simulink model "MPC_AVC"  (Simulink 8.5)
settings: Solver=ode5  StartTime=0.0  StopTime=4  FixedStep=dt  RelTol=1e-3
values from neighbouring files (symbols this model uses):
  A = F    [DMPC_AVC.m]    (also in Load_before.mat = [-209.443458109 -450.728478794 0 0 0 0 450.728478794 -209.44; Load_before_luan.mat = [-1.51362295222 -97.5366784553 0 0 0 0 95.8379605832 -0.9182)
  A_cons = [L_m;-L_m]    [DMPC_AVC.m]
  B = G    [DMPC_AVC.m]    (also in Load_before.mat = [-9.64474367822  2.65660382188; -7.76311006326  -5.616131872; Load_before_luan.mat = [-0.368065493108  -0.262854319087; -0.0702861565304  -0.0199)
  Bg = Bg(:,1:2)    [DMPC_AVC.m]
  C = H    [DMPC_AVC.m]    (also in Load_before.mat = [1.88477251669 -1.14284793707 5.77230310808 47.9525873536 -5; Load_before_luan.mat = [-15.8723139253 -1.67390261755 -0.939173865751 -0.9779387082)
  coefs = coefs(1,2:end)    [DMPC_AVC.m]
  dt = 0.00025    [DMPC_AVC.m]
  Hg = Bg(:,3)    [DMPC_AVC.m]
  L1 = dlqr(A',C',1e-5*eye(size(A)),1e-7)'    [DMPC_AVC.m]
  L2 = place(A',C',[0 0.1 -0.1 0.2 -0.2 0.3 -0.3 -0.4])    [DMPC_AVC.m]
  Lf = Kalman_Gain(A,C,Qf,Rf,Pf,Nsim,nout)    [DMPC_AVC.m]
  u_bound = [u_max;-u_min]    [DMPC_AVC.m]
undefined symbols (not defined in the file or in its folder): Ag, Cg, L_m, omega, psi
settings Model: Creator=Farhang  LastModifiedBy=p4wp4w
settings DebuggingCC: SolverPrmCheckMsg=warning  FcnCallInpInsideContextMsg=UseLocalSettings

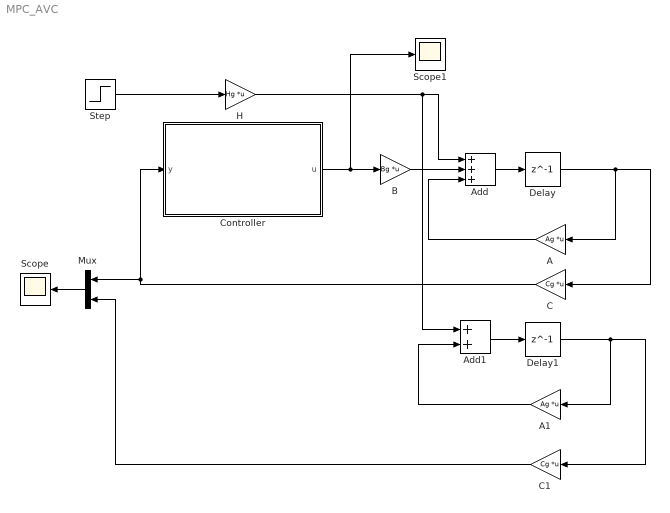
== system MPC_AVC ==
  A : Gain  Gain=Ag  Multiplication=Matrix(K*u)
  A1 : Gain  Gain=Ag  Multiplication=Matrix(K*u)
  Add : Sum  Inputs=+++
  Add1 : Sum
  B : Gain  Gain=Bg  Multiplication=Matrix(K*u)
  C : Gain  Gain=Cg  Multiplication=Matrix(K*u)
  C1 : Gain  Gain=Cg  Multiplication=Matrix(K*u)
  Controller : Subsystem
  Delay : Delay  DelayLength=1  InitialCondition=0
  Delay1 : Delay  DelayLength=1  InitialCondition=0
  H : Gain  Gain=Hg  Multiplication=Matrix(K*u)
  Mux : Mux  Inputs=2
  Scope : Scope
      settings: ShowLegends=on  YMin=-0.06  YMax=6.93889e-18
  Scope1 : Scope
      settings: ShowLegends=on  YMin=-0.0005  YMax=0.00055  SaveName=ScopeData2
  Step : Step  Time=2*dt  Before=1  After=0  SampleTime=0
  wires:
  Delay/1 -> A/1, C/1
  Controller/1(u) -> Scope1/1, B/1
  Add/1 -> Delay/1
  C/1 -> Mux/1, Controller/1(y)
  B/1 -> Add/2
  A/1 -> Add/3
  H/1 -> Add1/1, Add/1
  Step/1 -> H/1
  Delay1/1 -> C1/1, A1/1
  Add1/1 -> Delay1/1
  A1/1 -> Add1/2
  Mux/1 -> Scope/1
  C1/1 -> Mux/2

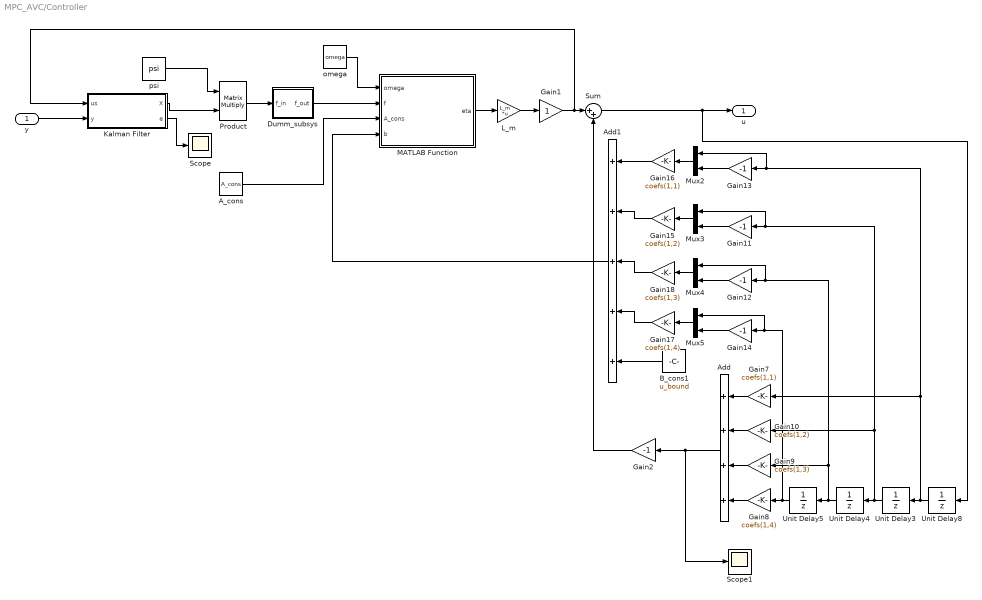
== system MPC_AVC/Controller ==
  y : Inport
  A_cons : Constant  Value=A_cons  SampleTime=dt
  Add : Sum  Inputs=++++
  Add1 : Sum  Inputs=+++++
  B_cons1 : Constant  Value=u_bound
  Dumm_subsys : Subsystem
  Gain1 : Gain
  Gain10 : Gain  Gain=coefs(1,2)
  Gain{2,11..14} (5 alike) : Gain  Gain=-1
  Gain15 : Gain  Gain=coefs(1,2)
  Gain16 : Gain  Gain=coefs(1,1)
  Gain17 : Gain  Gain=coefs(1,4)
  Gain18 : Gain  Gain=coefs(1,3)
  Gain7 : Gain  Gain=coefs(1,1)
  Gain8 : Gain  Gain=coefs(1,4)
  Gain9 : Gain  Gain=coefs(1,3)
  Kalman Filter : Subsystem  TreatAsAtomicUnit=on
  L_m : Gain  Gain=L_m  Multiplication=Matrix(K*u)
  MATLAB Function : MATLAB Function  TreatAsAtomicUnit=on
  Mux{2..5} (4 alike) : Mux  Inputs=2
  Product : Product  Multiplication=Matrix(*)  RndMeth=Zero
  Scope : Scope
      settings: YMin=-0.000155  YMax=-6.5e-05
  Scope1 : Scope
      settings: YMin=-0.00225  YMax=0.00225  SaveName=ScopeData3
  Sum : Sum  Inputs=|++
  Unit Delay{3..5,8} (4 alike) : UnitDelay  SampleTime=dt
  omega : Constant  Value=omega  SampleTime=dt
  psi : Constant  Value=psi  SampleTime=dt
  u : Outport
  wires:
  MATLAB Function/1(eta) -> L_m/1
  L_m/1 -> Gain1/1
  omega/1 -> MATLAB Function/1(omega)
  A_cons/1 -> MATLAB Function/3(A_cons)
  psi/1 -> Product/1
  y/1 -> Kalman Filter/2(y)
  Unit Delay8/1 -> Mux2/1, Gain13/1, Gain7/1, Unit Delay3/1
  Unit Delay3/1 -> Mux3/1, Gain11/1, Gain10/1, Unit Delay4/1
  Unit Delay5/1 -> Mux5/1, Gain14/1, Gain8/1
  Unit Delay4/1 -> Mux4/1, Gain12/1, Gain9/1, Unit Delay5/1
  Gain7/1 -> Add/1
  Gain9/1 -> Add/3
  Gain8/1 -> Add/4
  Gain13/1 -> Mux2/2
  Gain11/1 -> Mux3/2
  Gain12/1 -> Mux4/2
  Gain14/1 -> Mux5/2
  Mux2/1 -> Gain16/1
  Mux3/1 -> Gain15/1
  Mux4/1 -> Gain18/1
  Mux5/1 -> Gain17/1
  Gain16/1 -> Add1/1
  Gain15/1 -> Add1/2
  Gain18/1 -> Add1/3
  Gain17/1 -> Add1/4
  B_cons1/1 -> Add1/5
  Add1/1 -> MATLAB Function/4(b)
  Add/1 -> Scope1/1, Gain2/1
  Gain10/1 -> Add/2
  Product/1 -> Dumm_subsys/1(f_in)
  Dumm_subsys/1(f_out) -> MATLAB Function/2(f)
  Kalman Filter/1(X) -> Product/2
  Sum/1 -> Unit Delay8/1, u/1
  Kalman Filter/2(e) -> Scope/1
  Gain1/1 -> Sum/1, Kalman Filter/1(us)
  Gain2/1 -> Sum/2

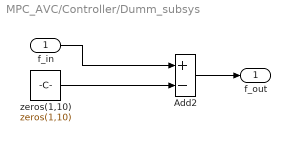
== system MPC_AVC/Controller/Dumm_subsys ==
  f_in : Inport
  Add2 : Sum  Inputs=+-
  zeros(1,10) : Constant  Value=zeros(1,10)  SampleTime=dt
  f_out : Outport
  wires:
  f_in/1 -> Add2/1
  Add2/1 -> f_out/1
  zeros(1,10)/1 -> Add2/2

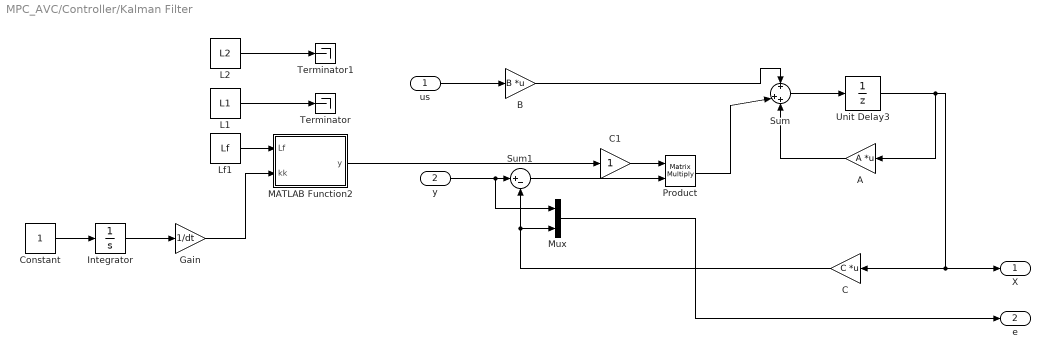
== system MPC_AVC/Controller/Kalman Filter ==
  us : Inport
  y : Inport  Port=2
  A : Gain  Gain=A  Multiplication=Matrix(K*u)
  B : Gain  Gain=B  Multiplication=Matrix(K*u)
  C : Gain  Gain=C  Multiplication=Matrix(K*u)
  C1 : Gain
  Constant : Constant
  Gain : Gain  Gain=1/dt
  Integrator : Integrator
  L1 : Constant  Value=L1
  L2 : Constant  Value=L2
  Lf1 : Constant  Value=Lf
  MATLAB Function2 : MATLAB Function  TreatAsAtomicUnit=on
  Mux : Mux  Inputs=2
  Product : Product  Multiplication=Matrix(*)  RndMeth=Zero
  Sum : Sum  Inputs=+|++
  Sum1 : Sum  Inputs=|+-
  Terminator : Terminator
  Terminator1 : Terminator
  Unit Delay3 : UnitDelay  SampleTime=dt
  X : Outport
  e : Outport  Port=2
  wires:
  Unit Delay3/1 -> A/1, X/1, C/1
  A/1 -> Sum/3
  Sum/1 -> Unit Delay3/1
  us/1 -> B/1
  B/1 -> Sum/1
  C/1 -> Mux/2, Sum1/2
  y/1 -> Mux/1, Sum1/1
  Sum1/1 -> Product/2
  Product/1 -> Sum/2
  Constant/1 -> Integrator/1
  Integrator/1 -> Gain/1
  Lf1/1 -> MATLAB Function2/1(Lf)
  Gain/1 -> MATLAB Function2/2(kk)
  L1/1 -> Terminator/1
  MATLAB Function2/1(y) -> C1/1
  L2/1 -> Terminator1/1
  C1/1 -> Product/1
  Mux/1 -> e/1

== matlab function Controller/MATLAB Function ==
  data: omega input double; eta output double; f input double; A_cons input double; b input double
function eta=QPomegaild(omega,f,A_cons,b)

[n1,m1]=size(A_cons);
% eta=-omega\f;
eta=-inv(omega)*f;
kk=0;
for i=1:n1
    if (A_cons(i,:)*eta>b(i)) 
        kk=kk+1;
    else
        kk=kk+0;
    end
end
if (kk==0)
    return
end
P=A_cons*(omega\A_cons');
d=(A_cons*(omega\f)+b);
[n,m]=size(d);
x_ini=zeros(n,m);
lambda=x_ini;
% al=10;
for km=1:38

%find tomegae elements in tomegae solution vector one by one
% km could be larger if tomegae Lagranger multiplier omegaas a slow
% convergence rate.
    lambda_p=lambda;
    for i=1:n
        w= P(i,:)*lambda-P(i,i)*lambda(i,1);
        w=w+d(i,1);
        la=-w/P(i,i);
        lambda(i,1)=max(0,la);
    end
    
    al=(lambda-lambda_p)'*(lambda-lambda_p);
    if (al<10e-8)
        break;
    end
 end
eta=-omega\f -omega\A_cons'*lambda;

== matlab function Controller/Kalman Filter/MATLAB Function2 ==
  data: y output double; Lf input double; kk input double
function y = fcn(Lf,kk)
%#codegen

kk = floor(kk)+1;

y = Lf(:,kk);
